simulink model "pv_static"  (R2025b)
settings: Solver=ode23tb  StartTime=0.0  StopTime=Tsim  MaxStep=5e-4  RelTol=1e-3
PreLoadFcn:
  | sb_grid_sim.init_load_internals('T1');
  | % --- PV-trip study defaults (overridden at sim time via params.model_vars) ---
  | P_pv=0.25*2405e6; f_trip=49.5; t_trip_delay=0.1;
undefined symbols (not defined in the file): CapC, dist_dP, dist_time, k_droop_f_g1, kt_hp, kt_lp, Lg_n1, M_g1, P_ref_g1, Rg_n1, Scc1, t_rh, theta_g0, Un1, Vpeak_g1, w_g1
libraries: spsControlledVoltageSourceLib x3, spsSeriesRLCBranchLib x3, spsGroundLib x2, spsThreePhaseParallelRLCLoadLib x1, spsThreePhaseParallelRLCBranchLib x1, spsThreePhaseVIMeasurementLib x1, spspowerguiLib x1
settings Model: Creator=madeleineneaves  LastModifiedBy=madeleineneaves

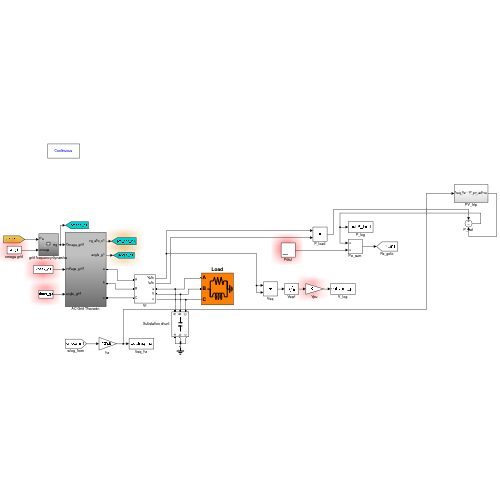
[thumbnail: Simulink's stored preview of the top-level diagram]
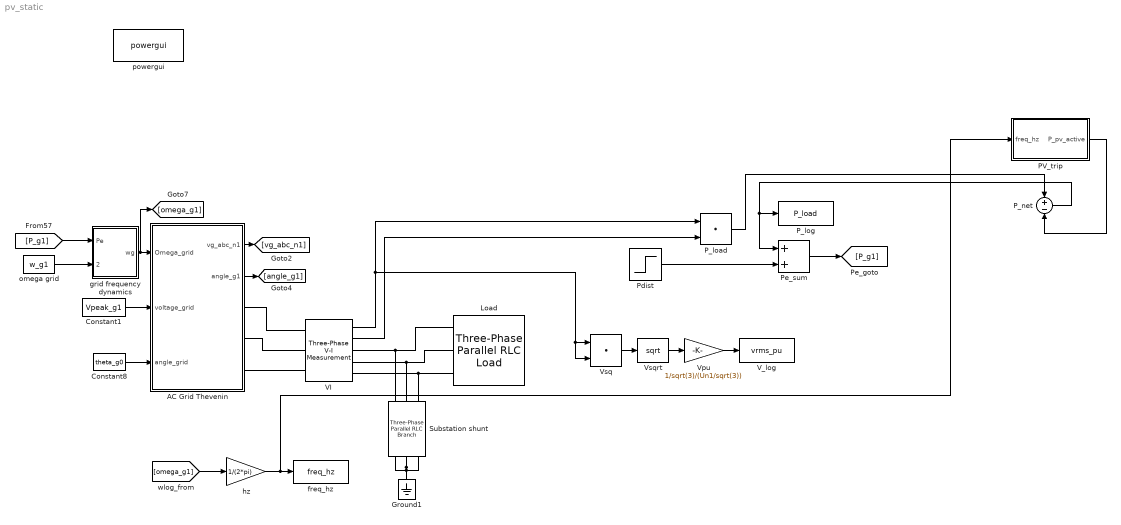
== system pv_static ==
  AC Grid Thevenin : Subsystem
  Constant1 : Constant  Value=Vpeak_g1
  Constant8 : Constant  Value=theta_g0
  Ground1 : spsGroundLib/Ground  LConnTagsString=a
  Load : spsThreePhaseParallelRLCLoadLib/Three-Phase Parallel RLC Load  LConnTagsString=A|B|C  Configuration=Y (grounded)  NominalVoltage=(220000)*1.00601  Vabc=[1e3 1e3 1e3]  Vabcp=[1e3 1e3 1e3]  NominalFrequency=50  UnbalancedPower=off  ActivePower=P_W  InductivePower=Q_var  CapacitivePower=0  Pabc=[10e3 9e3 11e3]  QLabc=[100 90 110]  QCabc=[100 90 110]  Pabcp=[10e3 9e3 11e3]  QLabcp=[100 90 110]  QCabcp=[100 90 110]  Measurements=None  LoadType=constant PQ
  PV_trip : Subsystem
  P_load : DotProduct  OutDataTypeStr=Inherit: Inherit via internal rule
  P_log : ToWorkspace  VariableName=P_load  SaveFormat=Timeseries  SampleTime=-1
  P_net : Sum  Inputs=+-
  Pdist : Step  Time=dist_time  After=dist_dP  SampleTime=0
  Pe_sum : Sum
  Substation shunt : spsThreePhaseParallelRLCBranchLib/Three-Phase Parallel RLC Branch  LConnTagsString=A|B|C  RConnTagsString=A|B|C  BranchType=C  Resistance=1  Inductance=1e-3  Capacitance=CapC  Measurements=None
  VI : spsThreePhaseVIMeasurementLib/Three-Phase V-I Measurement  VoltageMeasurement=phase-to-ground  SetLabelV=off  LabelV=Vabc  Vpu=off  VpuLL=off  CurrentMeasurement=yes  SetLabelI=off  LabelI=Iabc  Ipu=off  Pbase=100e6  Vbase=500e3  OutputType=Complex  PhasorSimulation=off  PSBequivalent=0
  V_log : ToWorkspace  VariableName=vrms_pu  SaveFormat=Timeseries  SampleTime=-1
  Vpu : Gain  Gain=1/sqrt(3)/(Un1/sqrt(3))
  Vsq : DotProduct  OutDataTypeStr=Inherit: Inherit via internal rule
  Vsqrt : Sqrt
  freq_hz : ToWorkspace  VariableName=freq_hz  SaveFormat=Timeseries  SampleTime=-1
  grid frequency dynamics : Subsystem
  hz : Gain  Gain=1/(2*pi)
  omega grid : Constant  Value=w_g1
  powergui : spspowerguiLib/powergui  Priority=1  SimulationMode=Continuous  SampleTime=50e-6  frequency=60  Iterations=50  frequencyindice=60  Pbase=100e6  ErrMax=1e-4  UnitsV=kV  UnitsW=MW  buscounter=0  FunctionMessages=off  echomessages=off  EnableUseOfTLC=off  CurrentSourceSwitches=off  DisableSnubberDevices=off  DisableRonSwitches=off  DisableVfSwitches=off  DisplayEquations=off  AutomaticDiscreteSolvers=off  SolverType=Tustin/Backward Euler (TBE)  Interpol=off  ExternalGateDelay=off  methode=off  Ts=100  x0status=blocks  SPID=on  SwTol=0  HookPort=off  NonlinearTolerance=1e-4  nMaxIteration=100  ContinueOnMaxIteration=off  RestoreLinks=warning  ResistiveCurrentMeasurement=off  Frange=[0:2:500]  Ylog=off  Xlog=on  ShowGrid=off  save=off  variable=ZData  structure=0  ZoomFFT=off  StartTime=0.0  cycles=1  DisplayStyle=1  fundamental=60  FreqAxis=off  MaxFrequency=1000  frequencyindicesteady=1  RmsSteady=1  display=off
  wires:
  AC Grid Thevenin/2(angle_g1) -> [angle_g1]
  Constant8/1 -> AC Grid Thevenin/3(angle_grid)
  Constant1/1 -> AC Grid Thevenin/2(voltage_grid)
  grid frequency dynamics/1(wg) -> [omega_g1], AC Grid Thevenin/1(Omega_grid)
  AC Grid Thevenin/1(vg_abc_n1) -> [vg_abc_n1]
  omega grid/1 -> grid frequency dynamics/2(omega)
  [P_g1] -> grid frequency dynamics/1(Pe)
  VI/1 -> Vsq/1, Vsq/2, P_load/1
  VI/2 -> P_load/2
  P_load/1 -> P_net/1
  Pdist/1 -> Pe_sum/2
  Pe_sum/1 -> [P_g1]
  [omega_g1] -> hz/1
  hz/1 -> PV_trip/1(freq_hz), freq_hz/1
  Vsq/1 -> Vsqrt/1
  Vsqrt/1 -> Vpu/1
  Vpu/1 -> V_log/1
  PV_trip/1(P_pv_active) -> P_net/2
  P_net/1 -> P_log/1, Pe_sum/1
  connections:
  AC Grid Thevenin/RConn1 -- VI/LConn1
  AC Grid Thevenin/RConn2 -- VI/LConn2
  AC Grid Thevenin/RConn3 -- VI/LConn3
  VI/RConn1 -- Substation shunt/LConn1 -- Load/LConn1
  VI/RConn2 -- Substation shunt/LConn2 -- Load/LConn2
  VI/RConn3 -- Load/LConn3 -- Substation shunt/LConn3
  Ground1/LConn1 -- Substation shunt/RConn2 -- Substation shunt/RConn3 -- Substation shunt/RConn1

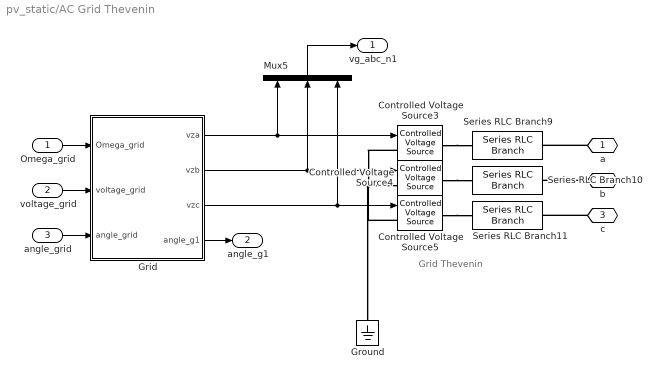
== system pv_static/AC Grid Thevenin ==
  note: Grid Thevenin
  Omega_grid : Inport
  voltage_grid : Inport  Port=2
  angle_grid : Inport  Port=3
  Controlled Voltage Source3 : spsControlledVoltageSourceLib/Controlled Voltage Source  Initialize=on  Source_Type=AC  Amplitude=0  Phase=0  Frequency=0  Measurements=None
  Controlled Voltage Source4 : spsControlledVoltageSourceLib/Controlled Voltage Source  Initialize=on  Source_Type=AC  Amplitude=0  Phase=0  Frequency=0  Measurements=None
  Controlled Voltage Source5 : spsControlledVoltageSourceLib/Controlled Voltage Source  Initialize=on  Source_Type=AC  Amplitude=0  Phase=0  Frequency=0  Measurements=None
  Grid : Subsystem
  Ground : spsGroundLib/Ground  LConnTagsString=a
  Mux5 : Mux  Inputs=3
  Series RLC Branch10 : spsSeriesRLCBranchLib/Series RLC Branch  LConnTagsString=__new0  RConnTagsString=__new0  BranchType=RL  Resistance=Rg_n1  Inductance=Lg_n1  SetiL0=off  InitialCurrent=0  Capacitance=0  Setx0=off  InitialVoltage=0  Measurements=None
  Series RLC Branch11 : spsSeriesRLCBranchLib/Series RLC Branch  LConnTagsString=__new0  RConnTagsString=__new0  BranchType=RL  Resistance=Rg_n1  Inductance=Lg_n1  SetiL0=off  InitialCurrent=0  Capacitance=0  Setx0=off  InitialVoltage=0  Measurements=None
  Series RLC Branch9 : spsSeriesRLCBranchLib/Series RLC Branch  LConnTagsString=__new0  RConnTagsString=__new0  BranchType=RL  Resistance=Rg_n1  Inductance=Lg_n1  SetiL0=off  InitialCurrent=0  Capacitance=0  Setx0=off  InitialVoltage=0  Measurements=None
  a : PMIOPort  Side=Right
  b : PMIOPort  Port=2  Side=Right
  c : PMIOPort  Port=3  Side=Right
  vg_abc_n1 : Outport
  angle_g1 : Outport  Port=2
  wires:
  Mux5/1 -> vg_abc_n1/1
  Grid/1(vza) -> Mux5/1, Controlled Voltage Source3/1
  Grid/2(vzb) -> Controlled Voltage Source4/1, Mux5/2
  Grid/3(vzc) -> Mux5/3, Controlled Voltage Source5/1
  voltage_grid/1 -> Grid/2(voltage_grid)
  Omega_grid/1 -> Grid/1(Omega_grid)
  angle_grid/1 -> Grid/3(angle_grid)
  Grid/4(angle_g1) -> angle_g1/1
  connections:
  Controlled Voltage Source3/LConn1 -- Controlled Voltage Source4/LConn1 -- Ground/LConn1 -- Controlled Voltage Source5/LConn1
  Controlled Voltage Source3/RConn1 -- Series RLC Branch9/LConn1
  a/RConn1 -- Series RLC Branch9/RConn1
  Controlled Voltage Source4/RConn1 -- Series RLC Branch10/LConn1
  c/RConn1 -- Series RLC Branch11/RConn1
  Controlled Voltage Source5/RConn1 -- Series RLC Branch11/LConn1
  b/RConn1 -- Series RLC Branch10/RConn1

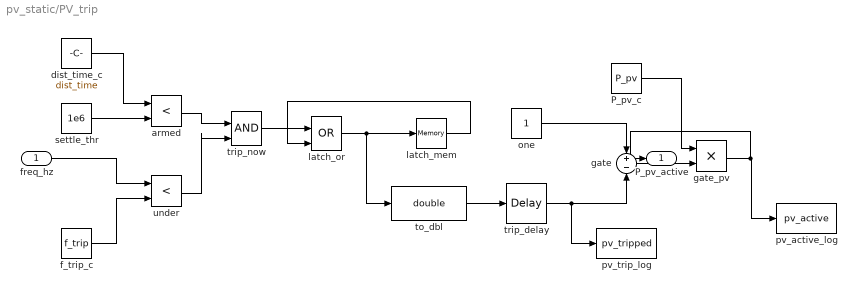
== system pv_static/PV_trip ==
  freq_hz : Inport
  P_pv_c : Constant  Value=P_pv
  armed : RelationalOperator  Operator=<  OutDataTypeStr=boolean  InputSameDT=off
  dist_time_c : Constant  Value=dist_time
  f_trip_c : Constant  Value=f_trip
  gate : Sum  Inputs=+-
  gate_pv : Product
  latch_mem : Memory
  latch_or : Logic  Operator=OR  IconShape=distinctive  AllPortsSameDT=off  OutDataTypeStr=boolean
  one : Constant
  pv_active_log : ToWorkspace  VariableName=pv_active  SaveFormat=Timeseries  SampleTime=-1
  pv_trip_log : ToWorkspace  VariableName=pv_tripped  SaveFormat=Timeseries  SampleTime=-1
  settle_thr : Constant  Value=1e6
  to_dbl : DataTypeConversion  OutDataTypeStr=double  SaturateOnIntegerOverflow=off  RndMeth=Floor
  trip_delay : TransportDelay  DelayTime=t_trip_delay
  trip_now : Logic  IconShape=distinctive  AllPortsSameDT=off  OutDataTypeStr=boolean
  under : RelationalOperator  Operator=<  OutDataTypeStr=boolean  InputSameDT=off
  P_pv_active : Outport
  wires:
  settle_thr/1 -> armed/2
  gate/1 -> gate_pv/2
  one/1 -> gate/1
  to_dbl/1 -> trip_delay/1
  freq_hz/1 -> under/1
  f_trip_c/1 -> under/2
  dist_time_c/1 -> armed/1
  armed/1 -> trip_now/1
  under/1 -> trip_now/2
  trip_now/1 -> latch_or/1
  latch_mem/1 -> latch_or/2
  latch_or/1 -> to_dbl/1, latch_mem/1
  trip_delay/1 -> pv_trip_log/1, gate/2
  P_pv_c/1 -> gate_pv/1
  gate_pv/1 -> pv_active_log/1, P_pv_active/1

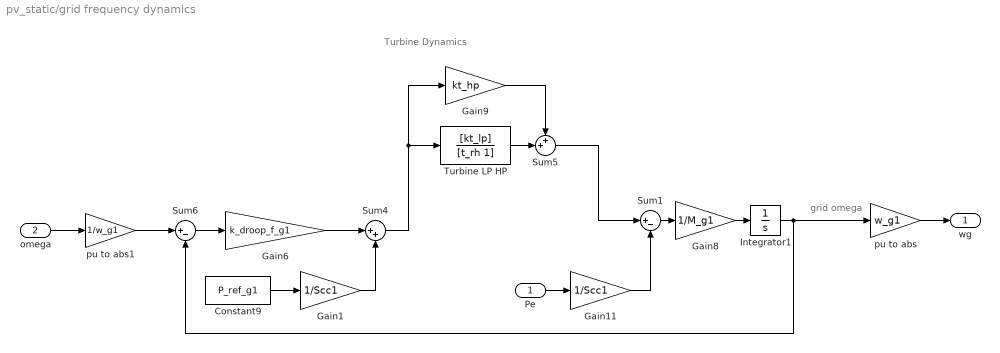
== system pv_static/grid frequency dynamics ==
  note: Turbine Dynamics
  note: grid omega
  Pe : Inport
  omega : Inport  Port=2
  Constant9 : Constant  Value=P_ref_g1
  Gain1 : Gain  Gain=1/Scc1
  Gain11 : Gain  Gain=1/Scc1
  Gain6 : Gain  Gain=k_droop_f_g1
  Gain8 : Gain  Gain=1/M_g1
  Gain9 : Gain  Gain=kt_hp
  Integrator1 : Integrator  InitialCondition=1
  Sum1 : Sum  Inputs=|+-
  Sum4 : Sum  Inputs=|++
  Sum5 : Sum  Inputs=++|
  Sum6 : Sum  Inputs=|+-
  Turbine LP HP : TransferFcn  Numerator=[kt_lp]  Denominator=[t_rh 1]
  pu to abs : Gain  Gain=w_g1
  pu to abs1 : Gain  Gain=1/w_g1
  wg : Outport
  wires:
  pu to abs1/1 -> Sum6/1
  Gain9/1 -> Sum5/1
  Sum6/1 -> Gain6/1
  Sum1/1 -> Gain8/1
  Integrator1/1 -> pu to abs/1, Sum6/2
  Gain11/1 -> Sum1/2
  Turbine LP HP/1 -> Sum5/2
  Sum4/1 -> Gain9/1, Turbine LP HP/1
  Gain6/1 -> Sum4/1
  Gain8/1 -> Integrator1/1
  Pe/1 -> Gain11/1
  pu to abs/1 -> wg/1
  Sum5/1 -> Sum1/1
  Gain1/1 -> Sum4/2
  omega/1 -> pu to abs1/1
  Constant9/1 -> Gain1/1

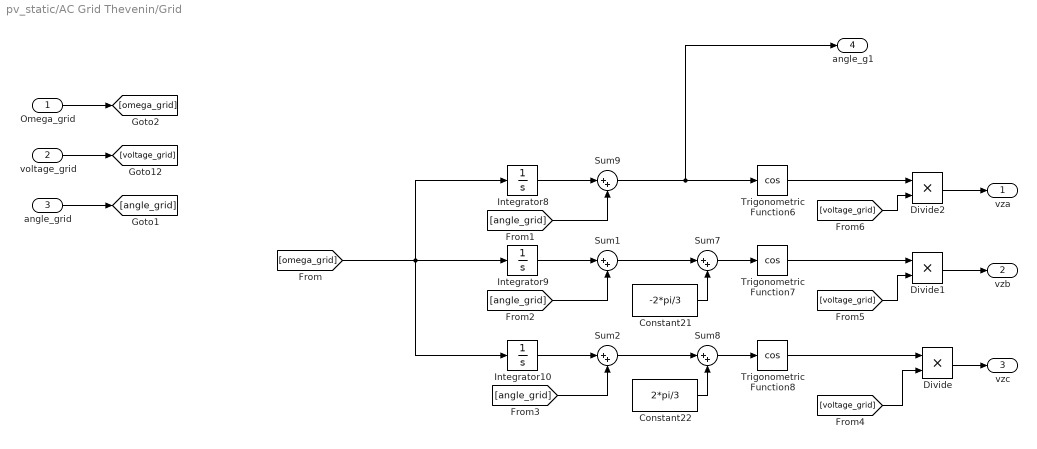
== system pv_static/AC Grid Thevenin/Grid ==
  Omega_grid : Inport
  voltage_grid : Inport  Port=2
  angle_grid : Inport  Port=3
  Constant21 : Constant  Value=-2*pi/3
  Constant22 : Constant  Value=2*pi/3
  Divide : Product  Inputs=**
  Divide1 : Product  Inputs=**
  Divide2 : Product  Inputs=**
  Integrator10 : Integrator
  Integrator8 : Integrator
  Integrator9 : Integrator
  Sum{1..2,7..9} (5 alike) : Sum  Inputs=|++
  Trigonometric Function6 : Trigonometry  Operator=cos
  Trigonometric Function7 : Trigonometry  Operator=cos
  Trigonometric Function8 : Trigonometry  Operator=cos
  vza : Outport  VectorParamsAs1DForOutWhenUnconnected=off
  vzb : Outport  Port=2  VectorParamsAs1DForOutWhenUnconnected=off
  vzc : Outport  Port=3  VectorParamsAs1DForOutWhenUnconnected=off
  angle_g1 : Outport  Port=4  VectorParamsAs1DForOutWhenUnconnected=off
  wires:
  Trigonometric Function8/1 -> Divide/1
  Trigonometric Function7/1 -> Divide1/1
  Sum9/1 -> angle_g1/1, Trigonometric Function6/1
  Constant22/1 -> Sum8/2
  Sum2/1 -> Sum8/1
  Constant21/1 -> Sum7/2
  Integrator8/1 -> Sum9/1
  Sum7/1 -> Trigonometric Function7/1
  [angle_grid] -> Sum9/2
  Sum1/1 -> Sum7/1
  Sum8/1 -> Trigonometric Function8/1
  Trigonometric Function6/1 -> Divide2/1
  [voltage_grid] -> Divide/2
  Divide/1 -> vzc/1
  Divide1/1 -> vzb/1
  Divide2/1 -> vza/1
  Integrator9/1 -> Sum1/1
  angle_grid/1 -> [angle_grid]
  voltage_grid/1 -> [voltage_grid]
  Omega_grid/1 -> [omega_grid]
  [omega_grid] -> Integrator10/1, Integrator8/1, Integrator9/1
  [angle_grid] -> Sum1/2
  Integrator10/1 -> Sum2/1
  [angle_grid] -> Sum2/2
  [voltage_grid] -> Divide1/2
  [voltage_grid] -> Divide2/2
